simulink model "Final_Project_Controller"  (R2017a)
settings: Solver=FixedStepAuto  StartTime=0.0  StopTime=inf  FixedStep=0.001  RelTol=1e-3  EnableMultiTasking=on
libraries: xpcquanserlib x5, slrtlib x3, dspswit3 x1
settings Model: SimulationMode=external  Creator=Venkatraman  LastModifiedBy=Noah Ruimveld
settings SolverCC: EnableConcurrentExecution=on
settings DataIOCC: LimitDataPoints=on  SaveFormat=Array
settings OptimizationCC: BlockReduction=off  OptimizeBlockIOStorage=off  BufferReuse=off  GlobalBufferReuse=off  ExpressionFolding=off  LocalBlockOutputs=off  LifeSpan=inf
settings DebuggingCC: SolverPrmCheckMsg=warning  SFUnexpectedBacktrackingDiag=warning  SFNoUnconditionalDefaultTransitionDiag=warning  SFExecutionAtInitializationDiag=none
settings HardwareCC: ProdBitPerPointer=32  ProdBitPerSizeT=32  ProdBitPerPtrDiffT=32  ProdLargestAtomicFloat=None  ProdWordSize=32  ProdLongLongMode=on  ProdHWDeviceType=Generic->32-bit x86 compatible  TargetBitPerPointer=64  TargetBitPerSizeT=64  TargetBitPerPtrDiffT=64  TargetLongLongMode=on  TargetIntDivRoundTo=Zero  TargetEndianess=LittleEndian  TargetWordSize=64  TargetHWDeviceType=MATLAB Host
settings ModelReferenceCC: PropagateSignalLabelsOutOfModel=off
settings RTWCC: SystemTargetFile=slrt.tlc  TemplateMakefile=slrt_default_tmf  Description=Simulink Real-Time  RTWVerbose=off  RTWCompilerOptimization=on
settings SimulinkRealTimeCC: GeneratePreprocessorConditionals=Disable all
settings ConfigComp: CovMetricSettings=dw  CovHtmlReporting=on  CovSaveCumulativeToWorkspaceVar=on  CovSaveSingleToWorkspaceVar=on  CovExternalEMLEnable=off  CovSFcnEnable=off

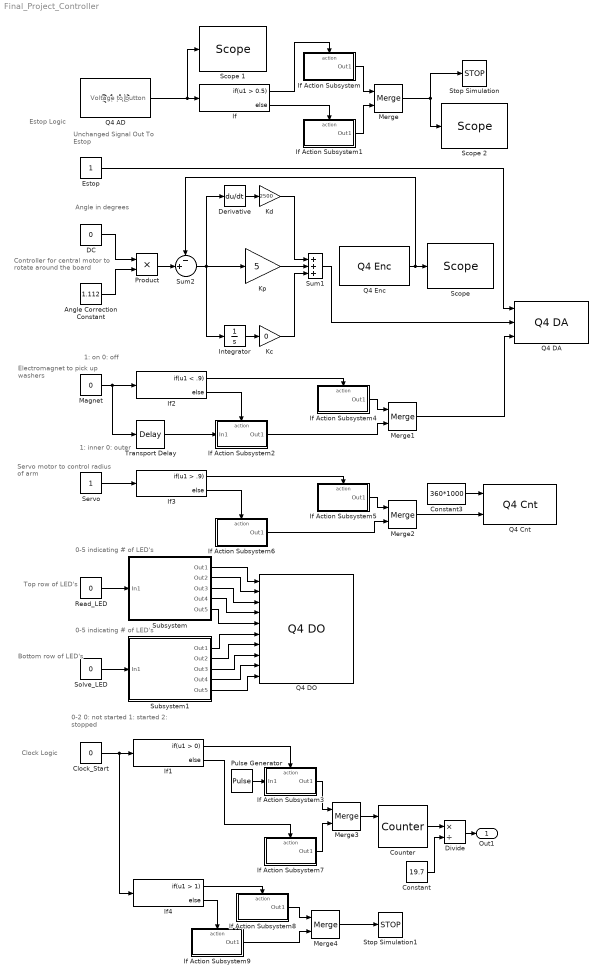
== system Final_Project_Controller ==
  note: 0-2
      | 0: not started
      | 1: started
      | 2: stopped
  note: Clock Logic
  note: Unchanged
      | Signal Out
      | To Estop
  note: 0-5
      | indicating
      | # of LED's
  note: Top row of
      | LED's
  note: Servo motor to
      | control radius
      | of arm
  note: Electromagnet
      | to pick up
      | washers
  note: Voltage to button
  note: 1: inner
      | 0: outer
  note: 1: on
      | 0: off
  note: Angle
      | in degrees
  note: Controller for
      | central motor
      | to rotate around
      | the board
  note: Estop
      | Logic
  note: Bottom row of
      | LED's
  note: 0-5
      | indicating
      | # of LED's
  Angle Correction Constant : Constant  Value=1.112
  Clock_Start : Constant  Value=0
  Constant : Constant  Value=19.7
  Constant3 : Constant  Value=360*1000
  Counter : dspswit3/Counter  Direction=Up  CountEvent=Rising edge  CounterSize=User defined  MaxCount=100000  InitialCount=0  Output=Count  HitValue=32  ResetInput=on  SamplesPerFrame=1  Ts=1  CntDtype=double  HitDtype=Logical
  DC : Constant  Value=0
  Derivative : Derivative
  Divide : Product  Inputs=*/
  Estop : Constant
  If : If  IfExpression=u1 > 0.5
  If Action Subsystem : Subsystem  TreatAsAtomicUnit=on
  If Action Subsystem1 : Subsystem  TreatAsAtomicUnit=on
  If Action Subsystem2 : Subsystem  TreatAsAtomicUnit=on
  If Action Subsystem3 : Subsystem  TreatAsAtomicUnit=on
  If Action Subsystem4 : Subsystem  TreatAsAtomicUnit=on
  If Action Subsystem5 : Subsystem  TreatAsAtomicUnit=on
  If Action Subsystem6 : Subsystem  TreatAsAtomicUnit=on
  If Action Subsystem7 : Subsystem  TreatAsAtomicUnit=on
  If Action Subsystem8 : Subsystem  TreatAsAtomicUnit=on
  If Action Subsystem9 : Subsystem  TreatAsAtomicUnit=on
  If1 : If
  If2 : If  IfExpression=u1 < .9
  If3 : If  IfExpression=u1 > .9
  If4 : If  IfExpression=u1 > 1
  Integrator : Integrator
  Kc : Gain  Gain=0
  Kd : Gain  Gain=2500
  Kp : Gain  Gain=5
  Magnet : Constant  Value=0
  Merge{,1..4} (5 alike) : Merge
  Product : Product
  Pulse Generator : DiscretePulseGenerator  PulseType=Time based  Period=1  PulseWidth=50  PhaseDelay=.1
  Q4 AD : xpcquanserlib/A//D/Q4 AD  channel=[2]  sampleTime=0.001  slot=-1
      settings: SourceProductName=Simulink Real-Time  SourceProductBaseCode=XP
  "Q4 Cnt " : xpcquanserlib/Counter/Q4 Cnt   channel=[1]  mode=[1]  showArm=[0]  reset=[1]  initLoCount=[0]  initHiCount=[0]  sampleTime=-1  slot=-1
      settings: SourceProductName=Simulink Real-Time  SourceProductBaseCode=XP
  "Q4 DA " : xpcquanserlib/D//A/Q4 DA   channel=[1 2 4]  range=[-5]  simul=off  reset=[1]  initValue=[0]  sampleTime=.001  slot=-1
      settings: SourceProductName=Simulink Real-Time  SourceProductBaseCode=XP
  "Q4 DO " : xpcquanserlib/Digital Output/Q4 DO   channel=[1 2 3 4 5 9 10 11 12 13]  reset=[1]  initValue=[0]  sampleTime=.001  slot=-1
      settings: SourceProductName=Simulink Real-Time  SourceProductBaseCode=XP
  "Q4 Enc " : xpcquanserlib/Incremental Encoder/Q4 Enc   channel=[2]  initialCount=[0]  prescale=[1]  quadrature=[1]  mode=[0]  synchronousIndex=[0]  indexPolarity=[0]  preserveCounts=[0]  sampleTime=.001  slot=-1
      settings: SourceProductName=Simulink Real-Time  SourceProductBaseCode=XP
  Read_LED : Constant  Value=0
  "Scope " : slrtlib/Displays and Logging/Scope   scopeno=1  scopetype=Target  autostart=on  viewmode=Graphical redraw  formatstr='%15.6f'  grid=on  ylimits=[0,0]  nosamples=250  noprepostsamples=0  interleave=1  triggermode=FreeRun  triggersignal=1  trigsignalfromport=off  triggerlevel=0.0  triggerslope=Either  triggerscope=1  triggersample=0  filename=data.dat  mode=Lazy  writesize=512  autorestart=off  dynamicfilemode=off  maxwritefilesize=512*1024^2
  Scope 1 : slrtlib/Displays and Logging/Scope   scopeno=3  scopetype=Target  autostart=on  viewmode=Graphical redraw  formatstr='%15.6f'  grid=on  ylimits=[0,0]  nosamples=250  noprepostsamples=0  interleave=1  triggermode=FreeRun  triggersignal=1  trigsignalfromport=off  triggerlevel=0.0  triggerslope=Either  triggerscope=1  triggersample=0  filename=data.dat  mode=Lazy  writesize=512  autorestart=off  dynamicfilemode=off  maxwritefilesize=512*1024^2
  Scope 2 : slrtlib/Displays and Logging/Scope   scopeno=2  scopetype=Target  autostart=on  viewmode=Graphical redraw  formatstr='%15.6f'  grid=on  ylimits=[0,0]  nosamples=250  noprepostsamples=0  interleave=1  triggermode=FreeRun  triggersignal=1  trigsignalfromport=off  triggerlevel=0.0  triggerslope=Either  triggerscope=1  triggersample=0  filename=data.dat  mode=Lazy  writesize=512  autorestart=off  dynamicfilemode=off  maxwritefilesize=512*1024^2
  Servo : Constant
  Solve_LED : Constant  Value=0
  Stop Simulation : Stop
  Stop Simulation1 : Stop
  Subsystem : Subsystem
  Subsystem1 : Subsystem
  Sum1 : Sum  Inputs=|+|+|+|
  Sum2 : Sum  Inputs=-+|
  Transport Delay : TransportDelay  DelayTime=.2
  Out1 : Outport  SignalName=Timer
  wires:
  Derivative/1 -> Kd/1
  Kd/1 -> Sum1/1
  Kc/1 -> Sum1/3
  Sum1/1 -> "Q4 DA "/2
  Kp/1 -> Sum1/2
  "Q4 Enc "/1 -> "Scope "/1, Sum2/1
  If Action Subsystem1/1(Out1) -> Merge/2
  Merge/1 -> Stop Simulation/1, Scope 2/1
  Q4 AD/1 -> Scope 1/1, If/1
  If/2 -> If Action Subsystem1/Action
  Estop/1 -> "Q4 DA "/1
  If Action Subsystem/1(Out1) -> Merge/1
  If/1 -> If Action Subsystem/Action
  Magnet/1 -> Transport Delay/1, If2/1
  If Action Subsystem2/1(Out1) -> Merge1/2
  If2/2 -> If Action Subsystem2/Action
  Merge1/1 -> "Q4 DA "/3
  If3/2 -> If Action Subsystem6/Action
  Servo/1 -> If3/1
  If3/1 -> If Action Subsystem5/Action
  If Action Subsystem4/1(Out1) -> Merge1/1
  Constant3/1 -> "Q4 Cnt "/1
  If Action Subsystem5/1(Out1) -> Merge2/1
  If Action Subsystem6/1(Out1) -> Merge2/2
  Merge2/1 -> "Q4 Cnt "/2
  If2/1 -> If Action Subsystem4/Action
  Transport Delay/1 -> If Action Subsystem2/1(In1)
  Read_LED/1 -> Subsystem/1(In1)
  DC/1 -> Product/1
  Angle Correction Constant/1 -> Product/2
  Integrator/1 -> Kc/1
  Sum2/1 -> Integrator/1, Derivative/1, Kp/1
  Product/1 -> Sum2/2
  Solve_LED/1 -> Subsystem1/1(In1)
  Subsystem/1(Out1) -> "Q4 DO "/1
  Subsystem/2(Out2) -> "Q4 DO "/2
  Subsystem/3(Out3) -> "Q4 DO "/3
  Subsystem/4(Out4) -> "Q4 DO "/4
  Subsystem/5(Out5) -> "Q4 DO "/5
  Subsystem1/5(Out5) -> "Q4 DO "/10
  Subsystem1/2(Out2) -> "Q4 DO "/7
  Subsystem1/4(Out4) -> "Q4 DO "/9
  Subsystem1/1(Out1) -> "Q4 DO "/6
  Subsystem1/3(Out3) -> "Q4 DO "/8
  Counter/1 -> Divide/1
  If1/1 -> If Action Subsystem3/Action
  If1/2 -> If Action Subsystem7/Action
  Merge3/1 -> Counter/1
  Pulse Generator/1 -> If Action Subsystem3/1(In1)
  If Action Subsystem7/1(Out1) -> Merge3/2
  If Action Subsystem3/1(Out1) -> Merge3/1
  Clock_Start/1 -> If4/1, If1/1
  Constant/1 -> Divide/2
  Divide/1 -> Out1/1
  If Action Subsystem9/1(Out1) -> Merge4/2
  If4/2 -> If Action Subsystem9/Action
  If4/1 -> If Action Subsystem8/Action
  If Action Subsystem8/1(Out1) -> Merge4/1
  Merge4/1 -> Stop Simulation1/1

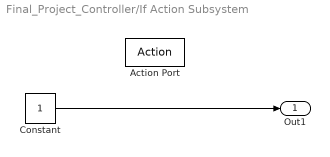
== system Final_Project_Controller/If Action Subsystem ==
  Action Port : ActionPort  ActionType=then
  Constant : Constant
  Out1 : Outport
  wires:
  Constant/1 -> Out1/1

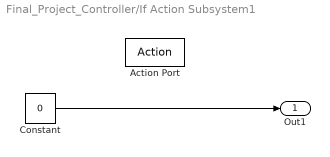
== system Final_Project_Controller/If Action Subsystem1 ==
  Action Port : ActionPort  ActionType=else
  Constant : Constant  Value=0
  Out1 : Outport
  wires:
  Constant/1 -> Out1/1

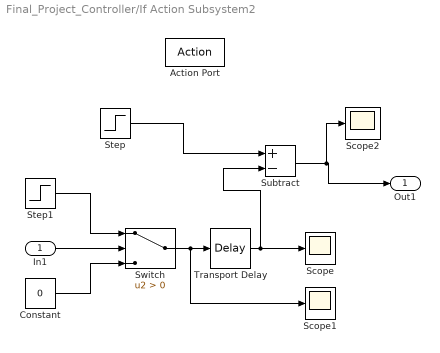
== system Final_Project_Controller/If Action Subsystem2 ==
  In1 : Inport
  Action Port : ActionPort  ActionType=else
  Constant : Constant  Value=0
  Scope : Scope
  Scope1 : Scope
  Scope2 : Scope
  Step : Step  After=10  SampleTime=0
  Step1 : Step  After=9.5  SampleTime=0
  Subtract : Sum  Inputs=+-
  Switch : Switch  Criteria=u2 > Threshold
  Transport Delay : TransportDelay  DelayTime=.5
  Out1 : Outport
  wires:
  In1/1 -> Switch/2
  Step/1 -> Subtract/1
  Subtract/1 -> Scope2/1, Out1/1
  Constant/1 -> Switch/3
  Transport Delay/1 -> Scope/1, Subtract/2
  Step1/1 -> Switch/1
  Switch/1 -> Scope1/1, Transport Delay/1

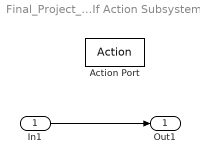
== system Final_Project_Controller/If Action Subsystem3 ==
  In1 : Inport
  Action Port : ActionPort  ActionType=then
  Out1 : Outport
  wires:
  In1/1 -> Out1/1

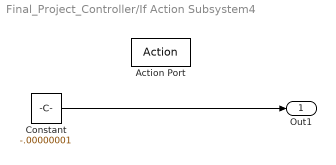
== system Final_Project_Controller/If Action Subsystem4 ==
  Action Port : ActionPort  ActionType=then
  Constant : Constant  Value=-.00000001
  Out1 : Outport
  wires:
  Constant/1 -> Out1/1

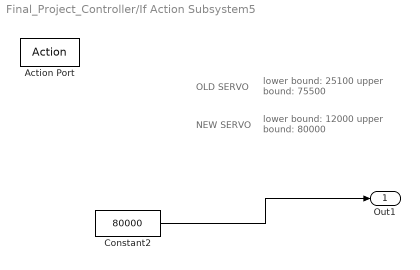
== system Final_Project_Controller/If Action Subsystem5 ==
  note: OLD SERVO
  note: lower bound: 25100
      | upper bound: 75500
  note: lower bound: 12000
      | upper bound: 80000
  note: NEW SERVO
  Action Port : ActionPort  ActionType=then
  Constant2 : Constant  Value=80000
  Out1 : Outport
  wires:
  Constant2/1 -> Out1/1

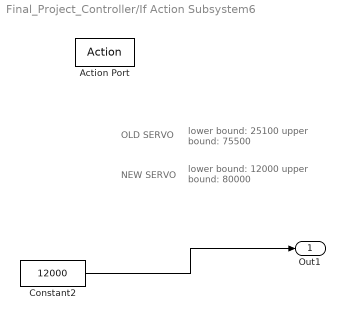
== system Final_Project_Controller/If Action Subsystem6 ==
  note: lower bound: 25100
      | upper bound: 75500
  note: NEW SERVO
  note: lower bound: 12000
      | upper bound: 80000
  note: OLD SERVO
  Action Port : ActionPort  ActionType=else
  Constant2 : Constant  Value=12000
  Out1 : Outport
  wires:
  Constant2/1 -> Out1/1

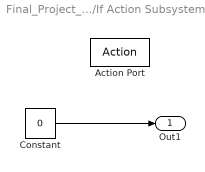
== system Final_Project_Controller/If Action Subsystem7 ==
  Action Port : ActionPort  ActionType=else
  Constant : Constant  Value=0
  Out1 : Outport
  wires:
  Constant/1 -> Out1/1

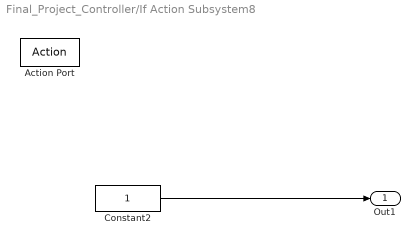
== system Final_Project_Controller/If Action Subsystem8 ==
  Action Port : ActionPort  ActionType=then
  Constant2 : Constant
  Out1 : Outport
  wires:
  Constant2/1 -> Out1/1

== system Final_Project_Controller/If Action Subsystem9 ==
  Action Port : ActionPort  ActionType=else
  Constant2 : Constant  Value=0
  Out1 : Outport
  wires:
  Constant2/1 -> Out1/1

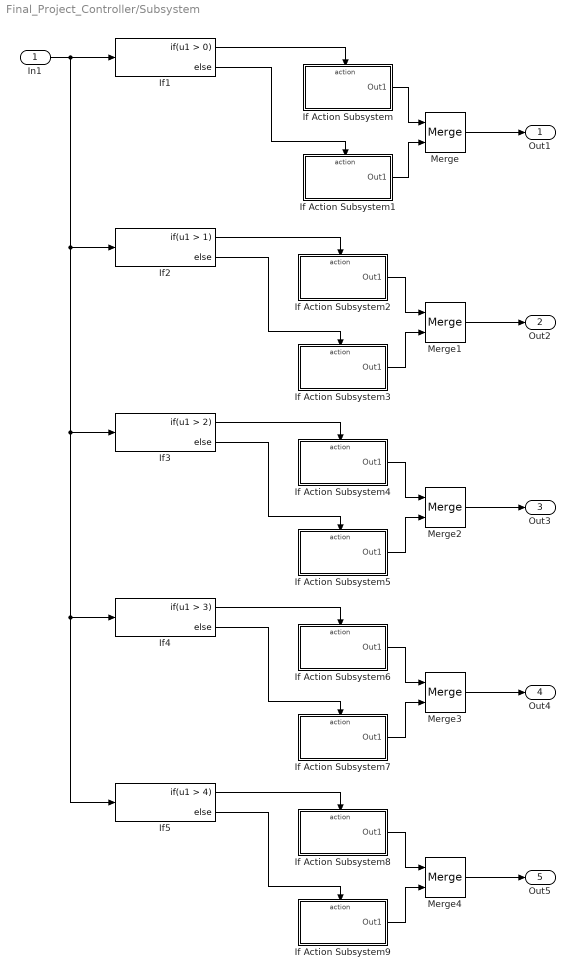
== system Final_Project_Controller/Subsystem ==
  In1 : Inport
  If Action Subsystem : Subsystem  TreatAsAtomicUnit=on
  If Action Subsystem1 : Subsystem  TreatAsAtomicUnit=on
  If Action Subsystem2 : Subsystem  TreatAsAtomicUnit=on
  If Action Subsystem3 : Subsystem  TreatAsAtomicUnit=on
  If Action Subsystem4 : Subsystem  TreatAsAtomicUnit=on
  If Action Subsystem5 : Subsystem  TreatAsAtomicUnit=on
  If Action Subsystem6 : Subsystem  TreatAsAtomicUnit=on
  If Action Subsystem7 : Subsystem  TreatAsAtomicUnit=on
  If Action Subsystem8 : Subsystem  TreatAsAtomicUnit=on
  If Action Subsystem9 : Subsystem  TreatAsAtomicUnit=on
  If1 : If
  If2 : If  IfExpression=u1 > 1
  If3 : If  IfExpression=u1 > 2
  If4 : If  IfExpression=u1 > 3
  If5 : If  IfExpression=u1 > 4
  Merge{,1..4} (5 alike) : Merge
  Out1 : Outport
  Out2 : Outport  Port=2
  Out3 : Outport  Port=3
  Out4 : Outport  Port=4
  Out5 : Outport  Port=5
  wires:
  In1/1 -> If5/1, If4/1, If3/1, If2/1, If1/1
  If5/1 -> If Action Subsystem8/Action
  If Action Subsystem8/1(Out1) -> Merge4/1
  If5/2 -> If Action Subsystem9/Action
  If Action Subsystem9/1(Out1) -> Merge4/2
  If Action Subsystem2/1(Out1) -> Merge1/1
  If Action Subsystem/1(Out1) -> Merge/1
  If Action Subsystem6/1(Out1) -> Merge3/1
  If4/1 -> If Action Subsystem6/Action
  If Action Subsystem7/1(Out1) -> Merge3/2
  If3/2 -> If Action Subsystem5/Action
  If3/1 -> If Action Subsystem4/Action
  If Action Subsystem4/1(Out1) -> Merge2/1
  If2/1 -> If Action Subsystem2/Action
  If Action Subsystem3/1(Out1) -> Merge1/2
  If2/2 -> If Action Subsystem3/Action
  If1/2 -> If Action Subsystem1/Action
  If4/2 -> If Action Subsystem7/Action
  If1/1 -> If Action Subsystem/Action
  If Action Subsystem5/1(Out1) -> Merge2/2
  If Action Subsystem1/1(Out1) -> Merge/2
  Merge/1 -> Out1/1
  Merge1/1 -> Out2/1
  Merge2/1 -> Out3/1
  Merge3/1 -> Out4/1
  Merge4/1 -> Out5/1

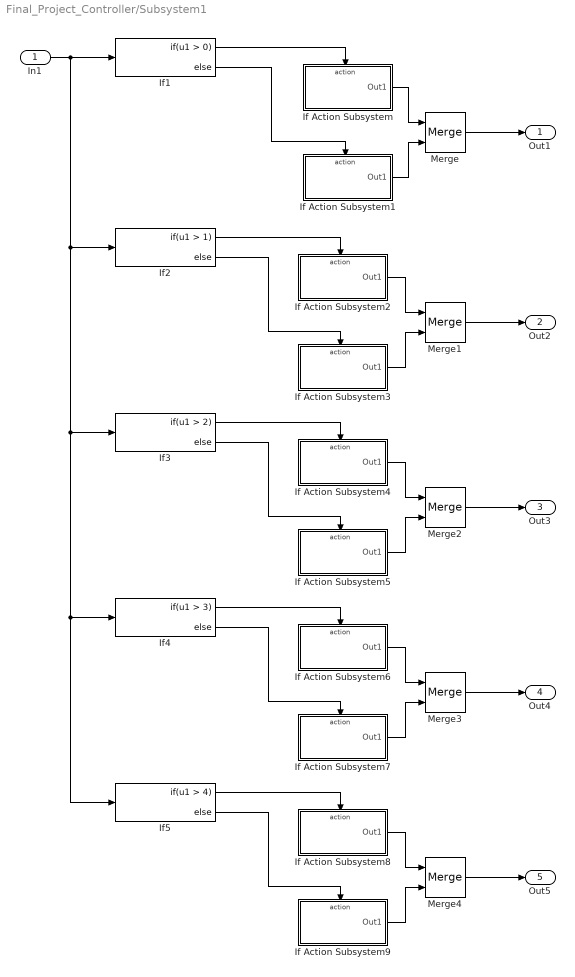
== system Final_Project_Controller/Subsystem1 ==
  In1 : Inport
  If Action Subsystem : Subsystem  TreatAsAtomicUnit=on
  If Action Subsystem1 : Subsystem  TreatAsAtomicUnit=on
  If Action Subsystem2 : Subsystem  TreatAsAtomicUnit=on
  If Action Subsystem3 : Subsystem  TreatAsAtomicUnit=on
  If Action Subsystem4 : Subsystem  TreatAsAtomicUnit=on
  If Action Subsystem5 : Subsystem  TreatAsAtomicUnit=on
  If Action Subsystem6 : Subsystem  TreatAsAtomicUnit=on
  If Action Subsystem7 : Subsystem  TreatAsAtomicUnit=on
  If Action Subsystem8 : Subsystem  TreatAsAtomicUnit=on
  If Action Subsystem9 : Subsystem  TreatAsAtomicUnit=on
  If1 : If
  If2 : If  IfExpression=u1 > 1
  If3 : If  IfExpression=u1 > 2
  If4 : If  IfExpression=u1 > 3
  If5 : If  IfExpression=u1 > 4
  Merge{,1..4} (5 alike) : Merge
  Out1 : Outport
  Out2 : Outport  Port=2
  Out3 : Outport  Port=3
  Out4 : Outport  Port=4
  Out5 : Outport  Port=5
  wires:
  In1/1 -> If5/1, If4/1, If3/1, If2/1, If1/1
  If5/1 -> If Action Subsystem8/Action
  If Action Subsystem8/1(Out1) -> Merge4/1
  If5/2 -> If Action Subsystem9/Action
  If Action Subsystem9/1(Out1) -> Merge4/2
  If Action Subsystem2/1(Out1) -> Merge1/1
  If Action Subsystem/1(Out1) -> Merge/1
  If Action Subsystem6/1(Out1) -> Merge3/1
  If4/1 -> If Action Subsystem6/Action
  If Action Subsystem7/1(Out1) -> Merge3/2
  If3/2 -> If Action Subsystem5/Action
  If3/1 -> If Action Subsystem4/Action
  If Action Subsystem4/1(Out1) -> Merge2/1
  If2/1 -> If Action Subsystem2/Action
  If Action Subsystem3/1(Out1) -> Merge1/2
  If2/2 -> If Action Subsystem3/Action
  If1/2 -> If Action Subsystem1/Action
  If4/2 -> If Action Subsystem7/Action
  If1/1 -> If Action Subsystem/Action
  If Action Subsystem5/1(Out1) -> Merge2/2
  If Action Subsystem1/1(Out1) -> Merge/2
  Merge/1 -> Out1/1
  Merge1/1 -> Out2/1
  Merge2/1 -> Out3/1
  Merge3/1 -> Out4/1
  Merge4/1 -> Out5/1

== system Final_Project_Controller/Subsystem/If Action Subsystem ==
  Action Port : ActionPort  ActionType=then
  Constant : Constant
  Out1 : Outport
  wires:
  Constant/1 -> Out1/1

== system Final_Project_Controller/Subsystem/If Action Subsystem1 ==
  Action Port : ActionPort  ActionType=else
  Constant : Constant  Value=0
  Out1 : Outport
  wires:
  Constant/1 -> Out1/1

== system Final_Project_Controller/Subsystem/If Action Subsystem2 ==
  Action Port : ActionPort  ActionType=then
  Constant : Constant
  Out1 : Outport
  wires:
  Constant/1 -> Out1/1

== system Final_Project_Controller/Subsystem/If Action Subsystem3 ==
  Action Port : ActionPort  ActionType=else
  Constant : Constant  Value=0
  Out1 : Outport
  wires:
  Constant/1 -> Out1/1

== system Final_Project_Controller/Subsystem/If Action Subsystem4 ==
  Action Port : ActionPort  ActionType=then
  Constant : Constant
  Out1 : Outport
  wires:
  Constant/1 -> Out1/1

== system Final_Project_Controller/Subsystem/If Action Subsystem5 ==
  Action Port : ActionPort  ActionType=else
  Constant : Constant  Value=0
  Out1 : Outport
  wires:
  Constant/1 -> Out1/1

== system Final_Project_Controller/Subsystem/If Action Subsystem6 ==
  Action Port : ActionPort  ActionType=then
  Constant : Constant
  Out1 : Outport
  wires:
  Constant/1 -> Out1/1

== system Final_Project_Controller/Subsystem/If Action Subsystem7 ==
  Action Port : ActionPort  ActionType=else
  Constant : Constant  Value=0
  Out1 : Outport
  wires:
  Constant/1 -> Out1/1

== system Final_Project_Controller/Subsystem/If Action Subsystem8 ==
  Action Port : ActionPort  ActionType=then
  Constant : Constant
  Out1 : Outport
  wires:
  Constant/1 -> Out1/1

== system Final_Project_Controller/Subsystem/If Action Subsystem9 ==
  Action Port : ActionPort  ActionType=else
  Constant : Constant  Value=0
  Out1 : Outport
  wires:
  Constant/1 -> Out1/1

== system Final_Project_Controller/Subsystem1/If Action Subsystem ==
  Action Port : ActionPort  ActionType=then
  Constant : Constant
  Out1 : Outport
  wires:
  Constant/1 -> Out1/1

== system Final_Project_Controller/Subsystem1/If Action Subsystem1 ==
  Action Port : ActionPort  ActionType=else
  Constant : Constant  Value=0
  Out1 : Outport
  wires:
  Constant/1 -> Out1/1

== system Final_Project_Controller/Subsystem1/If Action Subsystem2 ==
  Action Port : ActionPort  ActionType=then
  Constant : Constant
  Out1 : Outport
  wires:
  Constant/1 -> Out1/1

== system Final_Project_Controller/Subsystem1/If Action Subsystem3 ==
  Action Port : ActionPort  ActionType=else
  Constant : Constant  Value=0
  Out1 : Outport
  wires:
  Constant/1 -> Out1/1

== system Final_Project_Controller/Subsystem1/If Action Subsystem4 ==
  Action Port : ActionPort  ActionType=then
  Constant : Constant
  Out1 : Outport
  wires:
  Constant/1 -> Out1/1

== system Final_Project_Controller/Subsystem1/If Action Subsystem5 ==
  Action Port : ActionPort  ActionType=else
  Constant : Constant  Value=0
  Out1 : Outport
  wires:
  Constant/1 -> Out1/1

== system Final_Project_Controller/Subsystem1/If Action Subsystem6 ==
  Action Port : ActionPort  ActionType=then
  Constant : Constant
  Out1 : Outport
  wires:
  Constant/1 -> Out1/1

== system Final_Project_Controller/Subsystem1/If Action Subsystem7 ==
  Action Port : ActionPort  ActionType=else
  Constant : Constant  Value=0
  Out1 : Outport
  wires:
  Constant/1 -> Out1/1

== system Final_Project_Controller/Subsystem1/If Action Subsystem8 ==
  Action Port : ActionPort  ActionType=then
  Constant : Constant
  Out1 : Outport
  wires:
  Constant/1 -> Out1/1

== system Final_Project_Controller/Subsystem1/If Action Subsystem9 ==
  Action Port : ActionPort  ActionType=else
  Constant : Constant  Value=0
  Out1 : Outport
  wires:
  Constant/1 -> Out1/1
